simulink model "tesis_clasificador"  (R2013a)
settings: Solver=VariableStepDiscrete  StartTime=0.0  StopTime=100000  FixedStep=1  MaxStep=1  RelTol=1e-3
model workspace (MAT data in the model file):
  i = 1
values from neighbouring files (symbols this model uses):
  A_media = zeros(1,nic)    [entrenamiento_simulink.m]    (also in modelo_inicio.mat = 0; xe_y_t.mat = [0 0 0 0 0])
  invIC = transpose(IC_fastica)*inv(IC_fastica*transpose(IC_fastica))    [entrenamiento_simulink.m]    (also in modelo_inicio.mat = 0; xe_y_t.mat = [0 0 0 0 0 0 0 0 0 0 0 0 ... (1005 elements, 201x5)])
  rho = modelo.rho    [entrenamiento_simulink.m]
  sv = full(modelo.SVs)    [entrenamiento_simulink.m]
  sv_coef = modelo.sv_coef    [entrenamiento_simulink.m]
libraries: commfilt2 x1, simulink x1
settings Model: Creator=marcos  LastModifiedBy=marcos

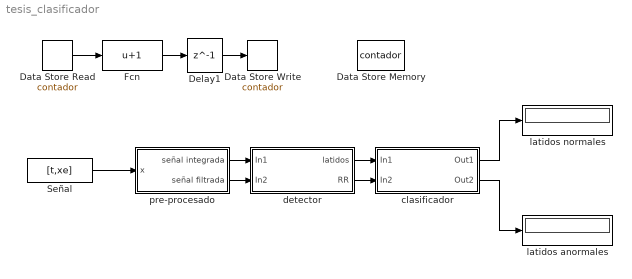
== system tesis_clasificador ==
  Data Store Memory : DataStoreMemory  DataStoreName=contador  ReadBeforeWriteMsg=warning  WriteAfterWriteMsg=warning  WriteAfterReadMsg=warning  InitialValue=1  OutDataTypeStr=double  Dimensions=1
  Data Store Read : DataStoreRead  DataStoreName=contador  SampleTime=1  DataStoreElements=contador
  Data Store Write : DataStoreWrite  DataStoreName=contador  SampleTime=1  DataStoreElements=contador
  Delay1 : Delay  DelayLength=1  InitialCondition=0  SampleTime=1
  Fcn : Fcn  Expr=u+1  SampleTime=1
  Señal : FromWorkspace  VariableName=[t,xe]  SampleTime=1
  clasificador : Subsystem  TreatAsAtomicUnit=on
  detector : Subsystem
  latidos anormales : Display
  latidos normales : Display
  pre-procesado : Subsystem
  wires:
  Señal/1 -> pre-procesado/1(x)
  pre-procesado/1(señal integrada) -> detector/1(In1)
  Fcn/1 -> Delay1/1
  Data Store Read/1 -> Fcn/1
  pre-procesado/2(señal filtrada) -> detector/2(In2)
  Delay1/1 -> Data Store Write/1
  detector/1(latidos) -> clasificador/1(In1)
  detector/2(RR) -> clasificador/2(In2)
  clasificador/1(Out1) -> latidos normales/1
  clasificador/2(Out2) -> latidos anormales/1

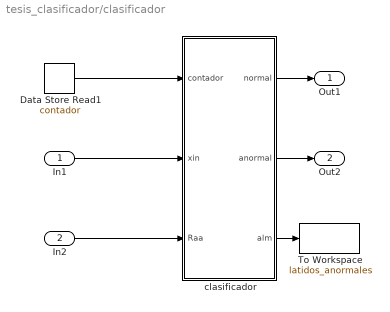
== system tesis_clasificador/clasificador ==
  In1 : Inport
  In2 : Inport  Port=2
  Data Store Read1 : DataStoreRead  DataStoreName=contador  SampleTime=1
  To Workspace : ToWorkspace  VariableName=latidos_anormales  SampleTime=-1
  clasificador : MATLAB Function  TreatAsAtomicUnit=on
  Out1 : Outport
  Out2 : Outport  Port=2
  wires:
  In1/1 -> clasificador/2(xin)
  clasificador/1(normal) -> Out1/1
  clasificador/2(anormal) -> Out2/1
  Data Store Read1/1 -> clasificador/1(contador)
  In2/1 -> clasificador/3(Raa)
  clasificador/3(alm) -> To Workspace/1

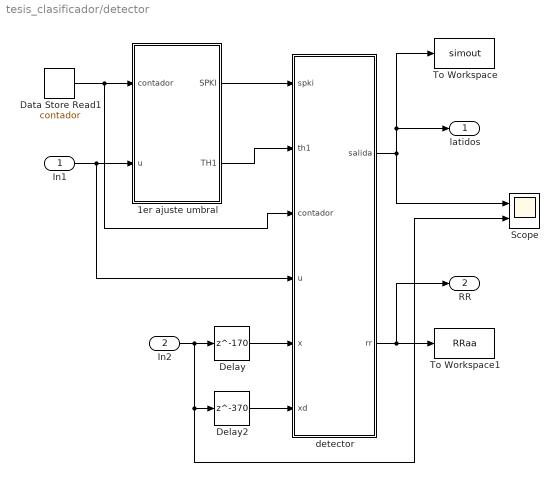
== system tesis_clasificador/detector ==
  In1 : Inport
  In2 : Inport  Port=2
  1er ajuste umbral : MATLAB Function  TreatAsAtomicUnit=on
  Data Store Read1 : DataStoreRead  DataStoreName=contador  SampleTime=1
  Delay : Delay  DelayLength=170  InitialCondition=0  SampleTime=1
  Delay2 : Delay  DelayLength=370  InitialCondition=0  SampleTime=1
  Scope : Scope  NumInputPorts=2
      settings: YMin=-40~-5  YMax=80~5  MaxDataPoints=10000
  To Workspace : ToWorkspace  VariableName=simout  SampleTime=-1
  To Workspace1 : ToWorkspace  VariableName=RRaa  SampleTime=1
  detector : MATLAB Function  TreatAsAtomicUnit=on
  latidos : Outport
  RR : Outport  Port=2
  wires:
  In1/1 -> detector/4(u), 1er ajuste umbral/2(u)
  Data Store Read1/1 -> detector/3(contador), 1er ajuste umbral/1(contador)
  1er ajuste umbral/1(SPKI) -> detector/1(spki)
  1er ajuste umbral/2(TH1) -> detector/2(th1)
  In2/1 -> Delay/1, Scope/2, Delay2/1
  detector/1(salida) -> latidos/1, To Workspace/1, Scope/1
  Delay2/1 -> detector/6(xd)
  Delay/1 -> detector/5(x)
  detector/2(rr) -> RR/1, To Workspace1/1

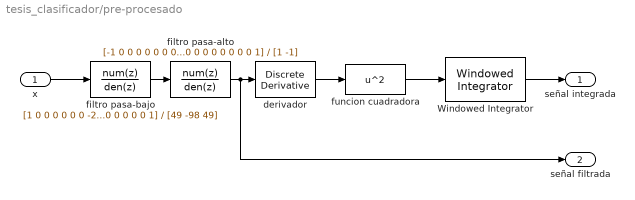
== system tesis_clasificador/pre-procesado ==
  x : Inport
  Windowed Integrator : commfilt2/Windowed Integrator  integperiod=64  roundingMode=Floor  overflowMode=off
  derivador : simulink/Discrete/Discrete Derivative  gainval=1.0  ICPrevScaledInput=0.0  InputProcessing=Inherited  OutMin=[]  OutMax=[]  OutDataType=fixdt(1, 16)  OutScaling=2^-10  DoSatur=off
  filtro pasa-alto : DiscreteFilter  Numerator=[-1 0 0 0 0 0 0 0 0 0 0 0 0 0 0 0 0 0 0 0 0 0 0 0 48 -48 0 0 0 0 0 0 0 0 0 0 0 0 0 0 0 0 0 0 0 0 0 0 1]  Denominator=[1 -1]
  filtro pasa-bajo : DiscreteFilter  Numerator=[1 0 0 0 0 0 0 -2 0 0 0 0 0 0 1]  Denominator=[49 -98 49]
  funcion cuadradora : Fcn  Expr=u^2
  señal integrada : Outport
  señal filtrada : Outport  Port=2
  wires:
  x/1 -> filtro pasa-bajo/1
  filtro pasa-bajo/1 -> filtro pasa-alto/1
  filtro pasa-alto/1 -> señal filtrada/1, derivador/1
  derivador/1 -> funcion cuadradora/1
  funcion cuadradora/1 -> Windowed Integrator/1
  Windowed Integrator/1 -> señal integrada/1

== matlab function tesis_clasificador/detector/detector ==
  data: spki input; th1 input; contador input; u input; salida output; x input; rr output; xd input
function [salida,rr]= fcn(spki,th1,contador,u,x,xd) 
%#codegen

%se definen las variables
persistent peak;
persistent TH1;
persistent SPKI;
persistent NPKI;
persistent bandera;     %bandera para buscar loma (1) o detectar qrs (2)
persistent guardar;     %bandera para guardar
persistent cuenta;
persistent sal;
persistent m_anterior;  %muestra anterior
persistent x_max;
persistent index;
persistent save;
persistent cuen;
persistent bkRR;
persistent relacion;
persistent pos_pico;

%se inician las variables
if isempty(peak)
    bkRR=[nan nan nan];
    peak=0;
    TH1=0;
    cuenta=1;
    guardar=0;
    sal=nan;
    m_anterior=-5;
    x_max=-10;
    bandera=1;
    index=nan;
    save=0;
    cuen=1;
    relacion=nan;
    pos_pico=nan;
end



%empiezo a detectar dsp del primer segundo 
if contador > 360

if isempty(SPKI)
    TH1=th1;
    NPKI=0;
    SPKI=spki;
end

switch (bandera)
    case {1} %Buscador de loma
        if u > m_anterior
            peak=u;
            bandera=2;
        end
        
    case {2} %Detector de QRS
        
        if u < (peak/2)

            if peak > TH1
            %actualiacion del umbral adaptativo (debido a la señal)
            SPKI=0.125*peak+0.875*SPKI;
            
            bandera=0;
            cuenta=1;
            guardar=1;
                        
            else
            %actualiacion del umbral adaptativo (debido al ruido)
            NPKI=0.125*peak+0.875*NPKI;
            bandera=1;
            end
            
        %actualiacion del umbral adaptativo
        TH1=NPKI+0.21*(SPKI-NPKI);
                
        
        elseif u > peak
        
        peak=u;
        
        end
    
    sal=nan;
    
end
        
%busco pico R
relacion=nan;

if guardar==1
    if cuenta <= 200
        if x > x_max
            index=cuenta;
            x_max=x;
            pos_pico=contador;
        end
        
    else
        %guardo los RR
        bkRR(3)=bkRR(2);
        bkRR(2)=bkRR(1);
        bkRR(1)=pos_pico;
        
        relacion=(bkRR(1)-bkRR(2))/(bkRR(2)-bkRR(3));
        
        save=1;
        x_max=-10;
        guardar=0;
        bandera=1;
        cuen=1;
        
    end

    cuenta=cuenta+1;
end

%guarda el latido centrado en R
if save==1
    if cuen >= (index-100) && cuen <= (index+100)
        
        sal=xd;
        relacion=(bkRR(1)-bkRR(2))/(bkRR(2)-bkRR(3));
        
    elseif cuen == (100+index)
        save=0;
        cuen=0;
        
    end

    cuen=cuen+1;
end

end
%guardo el valor actual para usarlo en el paso siguiente
m_anterior=u;

clasif=index;
t=TH1;
p=peak;
salida=sal;
rr=relacion;

== matlab function tesis_clasificador/detector/1er ajuste umbral ==
  data: contador input; u input; SPKI output; TH1 output
function [SPKI,TH1]= fcn(contador,u) 
%#codegen
persistent peak

if isempty(peak)
    peak=0;
end

if contador < 360

    if u > peak
        peak=u;
    end

end

%Ajuste de los umbrales de deteccion
%SPKI es el estimado del pico de señal
%NPKI es el estimado del pico de ruido
%THRESHOLD1 es el primer umbral aplicado 
%THRESHOLD2 es el segundo umbral aplicado.
SPKI=peak/2;
SPKI=0.125*peak+0.875*SPKI;

TH1=peak/4;

end

== matlab function tesis_clasificador/clasificador/clasificador ==
  data: contador input; xin input; Raa input; rho parameter; normal output; anormal output; sv parameter; sv_coef parameter; invIC parameter; A_media parameter; alm output
function [normal,anormal,alm]= fcn(contador,xin,Raa,rho,sv,sv_coef,invIC,A_media)
%#codegen

persistent lat_a;
persistent lat_n;
persistent num_svs;
persistent sv2;
persistent x2;
persistent cuenta;
persistent bandera;
persistent x;
persistent clasif;
persistent A;
persistent A_cl;
persistent K;
persistent busqueda;
persistent rr;
persistent f;
persistent almacenamiento;


if isempty(lat_a)
    lat_a=0;
    lat_n=0;
    cuenta=202;
    x=zeros(1,201);
    A=zeros(1,5);
    A_cl=zeros(1,5);
    clasif=0;
    busqueda=1;
    bandera=0;
    f=0;
    num_svs=size(sv, 1); %numero de SV
    sv2=sum(sv .* sv,2)'; % = norm(sv).^2
    K=zeros(1,num_svs);
    rr=nan;
    
end

if busqueda==1
    if isnan(xin)
       bandera=0;
       clasif=0;
    else
       bandera=1;
       cuenta=1;
       busqueda=0;
    end
end

f=0;

if bandera == 1
    if cuenta < 202
        x(cuenta)=xin;
        rr=Raa;
    else
        A=x*invIC;
   
        A_cl=A./A_media;
        
        bandera=0;
        clasif=1;
        
    end
    cuenta=cuenta+1;
end

almacenamiento=zeros(1,201)*nan;
if clasif==1
   
  x2 = sum([A_cl rr] .* [A_cl rr],2); % = norm(x).^2 
    
  K = exp(-0.3 * (x2*ones(1,num_svs) + ones(numel(1), 1)*sv2 - 2*[A_cl rr]*sv'));
         % for each sample i and for each support vector j -> y(i) = sum_j(sv_ceof(j) * exp(-gamma * norm(x(i)-sv(i)).^2)

  f= sign(K * sv_coef - rho);
  
  
  if f > 0
      lat_n=lat_n+1;
  elseif f < 0
      lat_a=lat_a+1;
      almacenamiento=x;
  end
  
  clasif=0;
  busqueda=1;
  %asd=3;
end


alm=almacenamiento;
normal=lat_n;
anormal=lat_a;
